simulink model "Subsystem"  (R2020b)
settings: Solver=VariableStepAuto  StartTime=0.0  StopTime=10.0  RelTol=1e-3
settings Model: Creator=Akarsh  LastModifiedBy=Akarsh
settings DataIOCC: SaveOutput=off  SaveTime=off

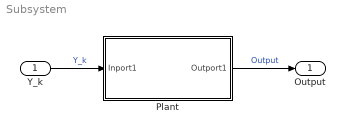
== system Subsystem ==
  Y_k : Inport  OutDataTypeStr=double  PortDimensions=1  SampleTime=0
  Plant : Subsystem
  Output : Outport  OutDataTypeStr=double  PortDimensions=1  SampleTime=0
  wires:
  Y_k/1 -> Plant/1(Inport1)  "Y_k"
  Plant/1(Outport1) -> Output/1  "Output"

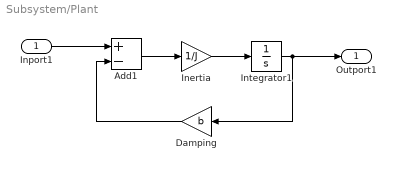
== system Subsystem/Plant ==
  Inport1 : Inport
  Add1 : Sum  Inputs=+-
  Damping : Gain  Gain=b  mask{b=20, Parameter2=0}
  Inertia : Gain  Gain=1/J  mask{J=100}
  Integrator1 : Integrator
  Outport1 : Outport
  wires:
  Inport1/1 -> Add1/1
  Damping/1 -> Add1/2
  Inertia/1 -> Integrator1/1
  Integrator1/1 -> Damping/1, Outport1/1
  Add1/1 -> Inertia/1
